simulink model "Four_PID_Ctrlr_for_DC_DC_Conv"  (R2024a)
settings: Solver=ode23tb  StartTime=0.0  StopTime=1  MaxStep=1e-4  RelTol=1e-3
libraries: spsSeriesRLCBranchLib x30, spsCurrentMeasurementLib x12, spsDCVoltageSourceLib x6, spsDiodeLib x6, spsIGBTLib x6, spsVoltageMeasurementLib x6, spspowerguiLib x5, slpidlib x1, simulink x1, sps_lib x1
settings Model: Creator=91889  LastModifiedBy=91889

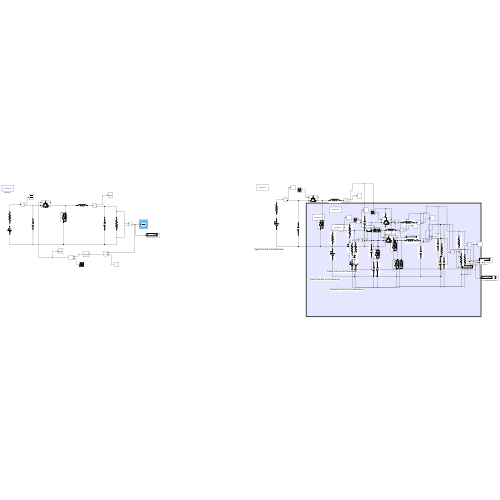
[thumbnail: Simulink's stored preview of the top-level diagram]
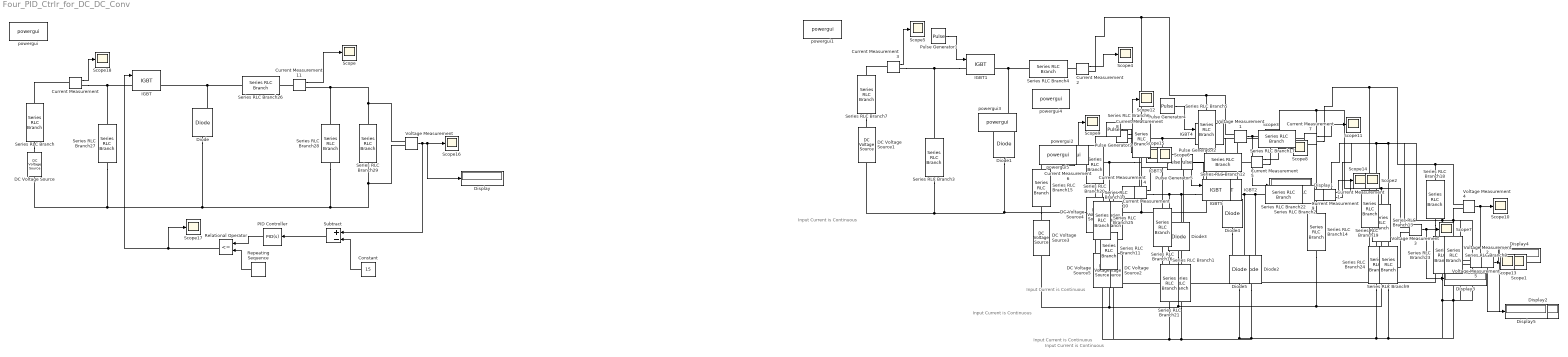
== system Four_PID_Ctrlr_for_DC_DC_Conv ==
  note: Input Current is Continuous
  note: Input Current is Continuous
  note: Input Current is Continuous
  note: Input Current is Continuous
  note: Input Current is Continuous
  Constant : Constant  Value=15
  Current Measurement{,1..11} (12 alike) : spsCurrentMeasurementLib/Current Measurement  PhasorSimulation=off  OutputType=Complex  PSBequivalent=0
  DC Voltage Source{,1..5} (6 alike) : spsDCVoltageSourceLib/DC Voltage Source  Amplitude=20  Measurements=None
  Diode{,1..5} (6 alike) : spsDiodeLib/Diode  Ron=0.001  Lon=0  Vf=0.8  IC=0  UseSnubber=0  Rs=500  Cs=250e-9  Measurements=on
  Display{,1..5} (6 alike) : Display
  IGBT : spsIGBTLib/IGBT  Ron=0.001  Lon=0  Vf=1  Tf=1e-6  Tt=2e-6  IC=0  Rs=1e5  Cs=inf  Measurements=on
  IGBT{1..5} (5 alike) : spsIGBTLib/IGBT  Ron=0.001  Lon=0  Vf=0  Tf=1e-6  Tt=2e-6  IC=0  Rs=1e5  Cs=inf  Measurements=on
  PID Controller : slpidlib/PID Controller  Controller=PID  Form=Parallel  TimeDomain=Continuous-time  UseExternalTs=off  SampleTime=-1  IntegratorMethod=Forward Euler  FilterMethod=Forward Euler  ControllerParametersSource=internal  P=12  I=25  UseKiTs=off  D=0  UseExternalDerivativeSource=off  N=100  UseFilter=on  TunerSelectOption=Transfer Function Based (PID Tuner App)  InitialConditionSource=internal  InitialConditionForIntegrator=0  InitialConditionForFilter=0  DifferentiatorICPrevScaledInput=0  ExternalReset=none  TrackingMode=off  Kt=1  LimitOutput=off  SatLimitsSource=internal  UpperSaturationLimit=inf  LowerSaturationLimit=-inf  LinearizeAsGain=on  AntiWindupMode=none  Kb=1  LimitIntegrator=off  UpperIntegratorSaturationLimit=inf  LowerIntegratorSaturationLimit=-inf  POutMin=[]  POutMax=[]  IOutMin=[]  IOutMax=[]  DOutMin=[]  DOutMax=[]  NOutMin=[]  NOutMax=[]  SumOutMin=[]  SumOutMax=[]  SaturationOutMin=[]  SaturationOutMax=[]  PParamMin=[]  PParamMax=[]  IParamMin=[]  IParamMax=[]  DParamMin=[]  DParamMax=[]  NParamMin=[]  NParamMax=[]  KbParamMin=[]  KbParamMax=[]  KtParamMin=[]  KtParamMax=[]  KbOutMin=[]  KbOutMax=[]  KtOutMin=[]  KtOutMax=[]  IntegratorOutMin=[]  IntegratorOutMax=[]  FilterOutMin=[]  FilterOutMax=[]  SumI1OutMin=[]  SumI1OutMax=[]  SumI2OutMin=[]  SumI2OutMax=[]  SumI3OutMin=[]  SumI3OutMax=[]  SumI4OutMin=[]  SumI4OutMax=[]  SumDOutMin=[]  SumDOutMax=[]  DifferentiatorOutMin=[]  DifferentiatorOutMax=[]  FilterDiffOutCoefMin=[]  FilterDiffOutCoefMax=[]  ReciprocalOutMin=[]  ReciprocalOutMax=[]  SumDenOutMin=[]  SumDenOutMax=[]  SumNumOutMin=[]  SumNumOutMax=[]  DivideOutMin=[]  DivideOutMax=[]  UdiffTsProdOutMin=[]  UdiffTsProdOutMax=[]  NTsProdOutMin=[]  NTsProdOutMax=[]  UintegralTsProdOutMin=[]  UintegralTsProdOutMax=[]  UngainTsProdOutMin=[]  UngainTsProdOutMax=[]  ClampingZeroOutDataTypeStr=Inherit: Inherit via back propagation  ClampingZeroOutMin=[]  ClampingZeroOutMax=[]  FilterDenConstantOutDataTypeStr=Inherit: Inherit via back propagation  FilterDenConstantOutMin=[]  FilterDenConstantOutMax=[]  PCopyOutDataTypeStr=Inherit: Inherit via back propagation  PCopyOutMin=[]  PCopyOutMax=[]  NCopyOutDataTypeStr=Inherit: Inherit via back propagation  NCopyOutMin=[]  NCopyOutMax=[]  IntegratorContinuousStateAttributes=''  IntegratorStateMustResolveToSignalObject=off  IntegratorRTWStateStorageClass=Auto  FilterContinuousStateAttributes=''  FilterStateMustResolveToSignalObject=off  FilterRTWStateStorageClass=Auto  ParallelPVariant=InternalParameters  IdealPVariant=Disabled  IVariant=InternalParameters  DVariant=InternalParameters  IntegratorVariant=Continuous  SatVariant=Disabled  AWVariant=Passthrough  PCopyVariant=Disabled  TRVariant=Disabled  FdbkBlocksVariant=Forward  IdealPFdbkVariant=Disabled  SatFdbkVariant=Disabled  DerivativeFilterVariant=ContFilter  NVariant=InternalParameters  NCopyVariant=Disabled  FilterICVariant=InternalICsFilter  IntegratorICVariant=InternalICs  ExternalResetVariant=Disabled  TRSumVariant=Passthrough  SumFdbkVariant=Disabled  SumVariant=Sum_PID  TsampFilterVariant=InternalTs  TsampNgainVariant=Passthrough  TsampIntegralVariant=Disabled_SignalSpec  ExternalSaturationOutDataTypeStr=Inherit: Same as second input  DerivativeSourceVariant=ErrorSignal
  Pulse Generator{1..5} (5 alike) : DiscretePulseGenerator  PulseType=Time based  Period=1/5000  PulseWidth=80
  Relational Operator : RelationalOperator  Operator=<=  OutDataTypeStr=boolean  RndMeth=Simplest  InputSameDT=off
  Repeating Sequence : simulink/Sources/Repeating Sequence  rep_seq_t=[0 1/5000]  rep_seq_y=[0 1]
  Scope{,1..18} (19 alike) : Scope
  Series RLC Branch : spsSeriesRLCBranchLib/Series RLC Branch  LConnTagsString=__new0  RConnTagsString=__new0  BranchType=R  Resistance=0.1  Inductance=1e-3  SetiL0=off  InitialCurrent=0  Capacitance=1e-6  Setx0=off  InitialVoltage=0  Measurements=None
  Series RLC Branch{1,3,11,16,21} (5 alike) : spsSeriesRLCBranchLib/Series RLC Branch  LConnTagsString=__new0  RConnTagsString=__new0  BranchType=C  Resistance=1  Inductance=1e-3  SetiL0=off  InitialCurrent=0  Capacitance=4800e-6  Setx0=off  InitialVoltage=0  Measurements=None
  Series RLC Branch{7,10,15,20,25} (5 alike) : spsSeriesRLCBranchLib/Series RLC Branch  LConnTagsString=__new0  RConnTagsString=__new0  BranchType=R  Resistance=0.1  Inductance=0.1e-3  SetiL0=on  InitialCurrent=0  Capacitance=1e-6  Setx0=off  InitialVoltage=0  Measurements=None
  Series RLC Branch{2,4,12,17,22} (5 alike) : spsSeriesRLCBranchLib/Series RLC Branch  LConnTagsString=__new0  RConnTagsString=__new0  BranchType=L  Resistance=1  Inductance=8e-3  SetiL0=on  InitialCurrent=0  Capacitance=1e-6  Setx0=off  InitialVoltage=0  Measurements=None
  Series RLC Branch{5,8,13,18,23} (5 alike) : spsSeriesRLCBranchLib/Series RLC Branch  LConnTagsString=__new0  RConnTagsString=__new0  BranchType=R  Resistance=10  Inductance=1e-3  SetiL0=off  InitialCurrent=0  Capacitance=1e-6  Setx0=off  InitialVoltage=0  Measurements=None
  Series RLC Branch{6,9,14,19,24} (5 alike) : spsSeriesRLCBranchLib/Series RLC Branch  LConnTagsString=__new0  RConnTagsString=__new0  BranchType=C  Resistance=1  Inductance=1e-3  SetiL0=off  InitialCurrent=0  Capacitance=5e-6  Setx0=off  InitialVoltage=0  Measurements=None
  Series RLC Branch26 : spsSeriesRLCBranchLib/Series RLC Branch  LConnTagsString=__new0  RConnTagsString=__new0  BranchType=L  Resistance=1  Inductance=8e-3  SetiL0=off  InitialCurrent=0  Capacitance=1e-6  Setx0=off  InitialVoltage=0  Measurements=None
  Series RLC Branch27 : spsSeriesRLCBranchLib/Series RLC Branch  LConnTagsString=__new0  RConnTagsString=__new0  BranchType=C  Resistance=0.1  Inductance=1e-3  SetiL0=off  InitialCurrent=0  Capacitance=4800e-6  Setx0=off  InitialVoltage=0  Measurements=None
  Series RLC Branch28 : spsSeriesRLCBranchLib/Series RLC Branch  LConnTagsString=__new0  RConnTagsString=__new0  BranchType=C  Resistance=0.1  Inductance=1e-3  SetiL0=off  InitialCurrent=0  Capacitance=5e-6  Setx0=off  InitialVoltage=0  Measurements=None
  Series RLC Branch29 : spsSeriesRLCBranchLib/Series RLC Branch  LConnTagsString=__new0  RConnTagsString=__new0  BranchType=R  Resistance=10  Inductance=1e-3  SetiL0=off  InitialCurrent=0  Capacitance=5e-6  Setx0=off  InitialVoltage=0  Measurements=None
  Subtract : Sum  Inputs=+-
  Voltage Measurement{,1..5} (6 alike) : spsVoltageMeasurementLib/Voltage Measurement  PhasorSimulation=off  OutputType=Complex  PSBequivalent=0
  powergui : sps_lib/powergui  Priority=1  SimulationMode=Continuous  SampleTime=50e-6  frequency=60  Iterations=50  frequencyindice=0  Pbase=100e6  ErrMax=1e-4  UnitsV=kV  UnitsW=MW  buscounter=0  FunctionMessages=off  echomessages=off  EnableUseOfTLC=off  CurrentSourceSwitches=off  DisableSnubberDevices=off  DisableRonSwitches=off  DisableVfSwitches=off  DisplayEquations=off  AutomaticDiscreteSolvers=off  SolverType=Tustin/Backward Euler (TBE)  Interpol=off  ExternalGateDelay=off  methode=off  Ts=100  x0status=blocks  SPID=on  SwTol=0  HookPort=off  NonlinearTolerance=1e-4  nMaxIteration=100  ContinueOnMaxIteration=off  RestoreLinks=warning  ResistiveCurrentMeasurement=off  Frange=[0:2:500]  Ylog=off  Xlog=on  ShowGrid=off  save=off  variable=ZData  structure=0  ZoomFFT=off  StartTime=0.0  cycles=1  DisplayStyle=1  fundamental=60  FreqAxis=off  MaxFrequency=1000  frequencyindicesteady=1  RmsSteady=1  display=off
  powergui{1..5} (5 alike) : spspowerguiLib/powergui  Priority=1  SimulationMode=Continuous  SampleTime=50e-6  frequency=60  Iterations=50  frequencyindice=0  Pbase=100e6  ErrMax=1e-4  UnitsV=kV  UnitsW=MW  buscounter=0  FunctionMessages=off  echomessages=off  EnableUseOfTLC=off  CurrentSourceSwitches=off  DisableSnubberDevices=off  DisableRonSwitches=off  DisableVfSwitches=off  DisplayEquations=off  AutomaticDiscreteSolvers=off  SolverType=Tustin/Backward Euler (TBE)  Interpol=off  ExternalGateDelay=off  methode=off  Ts=100  x0status=blocks  SPID=on  SwTol=0  HookPort=off  NonlinearTolerance=1e-4  nMaxIteration=100  ContinueOnMaxIteration=off  RestoreLinks=warning  ResistiveCurrentMeasurement=off  Frange=[0:2:500]  Ylog=off  Xlog=on  ShowGrid=off  save=off  variable=ZData  structure=0  ZoomFFT=off  StartTime=0.0  cycles=1  DisplayStyle=1  fundamental=60  FreqAxis=off  MaxFrequency=1000  frequencyindicesteady=1  RmsSteady=1  display=off
  wires:
  Pulse Generator1/1 -> IGBT1/1
  Voltage Measurement1/1 -> Display1/1, Scope3/1
  Current Measurement2/1 -> Scope4/1
  Current Measurement3/1 -> Scope5/1
  Pulse Generator2/1 -> IGBT2/1
  Voltage Measurement2/1 -> Display2/1, Scope1/1
  Current Measurement1/1 -> Scope2/1
  Current Measurement4/1 -> Scope6/1
  Pulse Generator3/1 -> IGBT3/1
  Voltage Measurement3/1 -> Display3/1, Scope7/1
  Current Measurement5/1 -> Scope8/1
  Current Measurement6/1 -> Scope9/1
  Pulse Generator4/1 -> IGBT4/1
  Voltage Measurement4/1 -> Display4/1, Scope10/1
  Current Measurement7/1 -> Scope11/1
  Current Measurement8/1 -> Scope12/1
  Pulse Generator5/1 -> IGBT5/1
  Voltage Measurement5/1 -> Display5/1, Scope13/1
  Current Measurement9/1 -> Scope14/1
  Current Measurement10/1 -> Scope15/1
  Current Measurement11/1 -> Scope/1
  Voltage Measurement/1 -> Subtract/1, Display/1, Scope16/1
  Current Measurement/1 -> Scope18/1
  Constant/1 -> Subtract/2
  Subtract/1 -> PID Controller/1
  PID Controller/1 -> Relational Operator/1
  Repeating Sequence/1 -> Relational Operator/2
  Relational Operator/1 -> Scope17/1, IGBT/1
  connections:
  Series RLC Branch4/LConn1 -- IGBT1/RConn1 -- Diode1/RConn1
  Series RLC Branch5/LConn1 -- Current Measurement2/RConn1 -- Series RLC Branch6/LConn1 -- Voltage Measurement1/LConn1
  IGBT1/LConn1 -- Current Measurement3/RConn1 -- Series RLC Branch3/LConn1
  DC Voltage Source1/LConn1 -- Series RLC Branch6/RConn1 -- Series RLC Branch5/RConn1 -- Voltage Measurement1/LConn2 -- Diode1/LConn1 -- Series RLC Branch3/RConn1
  Current Measurement2/LConn1 -- Series RLC Branch4/RConn1
  Series RLC Branch7/LConn1 -- Current Measurement3/LConn1
  Series RLC Branch7/RConn1 -- DC Voltage Source1/RConn1
  Series RLC Branch2/LConn1 -- IGBT2/RConn1 -- Diode2/RConn1
  Series RLC Branch8/LConn1 -- Current Measurement1/RConn1 -- Series RLC Branch9/LConn1 -- Voltage Measurement2/LConn1
  IGBT2/LConn1 -- Current Measurement4/RConn1 -- Series RLC Branch1/LConn1
  DC Voltage Source2/LConn1 -- Series RLC Branch9/RConn1 -- Series RLC Branch8/RConn1 -- Voltage Measurement2/LConn2 -- Diode2/LConn1 -- Series RLC Branch1/RConn1
  Current Measurement1/LConn1 -- Series RLC Branch2/RConn1
  Series RLC Branch10/LConn1 -- Current Measurement4/LConn1
  Series RLC Branch10/RConn1 -- DC Voltage Source2/RConn1
  Series RLC Branch12/LConn1 -- IGBT3/RConn1 -- Diode3/RConn1
  Series RLC Branch13/LConn1 -- Current Measurement5/RConn1 -- Series RLC Branch14/LConn1 -- Voltage Measurement3/LConn1
  IGBT3/LConn1 -- Current Measurement6/RConn1 -- Series RLC Branch11/LConn1
  DC Voltage Source3/LConn1 -- Series RLC Branch14/RConn1 -- Series RLC Branch13/RConn1 -- Voltage Measurement3/LConn2 -- Diode3/LConn1 -- Series RLC Branch11/RConn1
  Series RLC Branch15/LConn1 -- Current Measurement6/LConn1
  Series RLC Branch15/RConn1 -- DC Voltage Source3/RConn1
  Current Measurement5/LConn1 -- Series RLC Branch12/RConn1
  Series RLC Branch17/LConn1 -- IGBT4/RConn1 -- Diode4/RConn1
  Series RLC Branch18/LConn1 -- Current Measurement7/RConn1 -- Series RLC Branch19/LConn1 -- Voltage Measurement4/LConn1
  IGBT4/LConn1 -- Current Measurement8/RConn1 -- Series RLC Branch16/LConn1
  DC Voltage Source4/LConn1 -- Series RLC Branch19/RConn1 -- Series RLC Branch18/RConn1 -- Voltage Measurement4/LConn2 -- Diode4/LConn1 -- Series RLC Branch16/RConn1
  Series RLC Branch20/RConn1 -- DC Voltage Source4/RConn1
  Series RLC Branch20/LConn1 -- Current Measurement8/LConn1
  Current Measurement7/LConn1 -- Series RLC Branch17/RConn1
  Series RLC Branch22/LConn1 -- IGBT5/RConn1 -- Diode5/RConn1
  Series RLC Branch23/LConn1 -- Current Measurement9/RConn1 -- Series RLC Branch24/LConn1 -- Voltage Measurement5/LConn1
  IGBT5/LConn1 -- Current Measurement10/RConn1 -- Series RLC Branch21/LConn1
  DC Voltage Source5/LConn1 -- Series RLC Branch24/RConn1 -- Series RLC Branch23/RConn1 -- Voltage Measurement5/LConn2 -- Diode5/LConn1 -- Series RLC Branch21/RConn1
  Series RLC Branch25/RConn1 -- DC Voltage Source5/RConn1
  Series RLC Branch25/LConn1 -- Current Measurement10/LConn1
  Current Measurement9/LConn1 -- Series RLC Branch22/RConn1
  Series RLC Branch/RConn1 -- DC Voltage Source/RConn1
  Current Measurement/LConn1 -- Series RLC Branch/LConn1
  Current Measurement/RConn1 -- IGBT/LConn1 -- Series RLC Branch27/LConn1
  Diode/RConn1 -- Series RLC Branch26/LConn1 -- IGBT/RConn1
  Current Measurement11/LConn1 -- Series RLC Branch26/RConn1
  Series RLC Branch28/LConn1 -- Voltage Measurement/LConn1 -- Series RLC Branch29/LConn1 -- Current Measurement11/RConn1
  Series RLC Branch29/RConn1 -- Voltage Measurement/LConn2 -- Series RLC Branch28/RConn1 -- Diode/LConn1 -- Series RLC Branch27/RConn1 -- DC Voltage Source/LConn1
